simulink library "generallib"  (R2024b)
settings: Solver=VariableStepAuto  StartTime=0.0  StopTime=10.0  RelTol=1e-3
Description:
  | Simulink library with commonly used blocks for
  | Robotics, Vision and Control - 3rd Edition
settings Model: Creator=rpill  LastModifiedBy=pic
settings SolverCC: MaxZcPerStep=1
settings DebuggingCC: UnconnectedInputMsg=warning  UnconnectedOutputMsg=warning  UnconnectedLineMsg=warning
settings ModelReferenceCC: EnableRefExpFcnMdlSchedulingChecks=on
settings RTWCC: GPUComputeCapability=3.5  DLArmComputeVersion=19.05

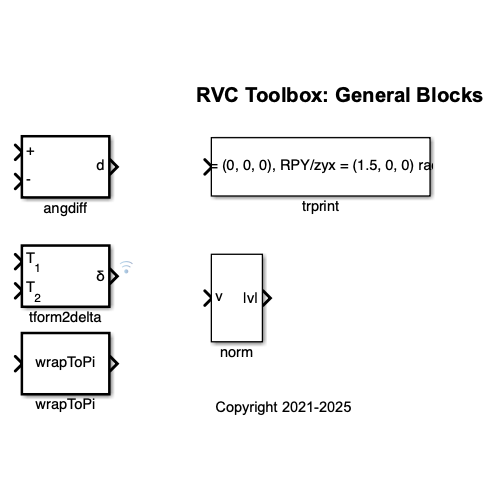
[thumbnail: Simulink's stored preview of the top-level diagram]
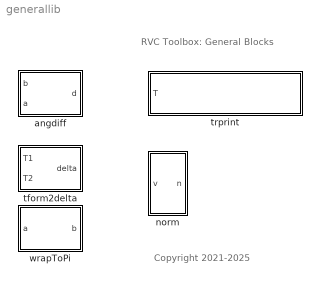
== system generallib ==
  note: Copyright 2021-2025
  note: RVC Toolbox: General Blocks
  angdiff : MATLAB Function  TreatAsAtomicUnit=on
  norm : Subsystem
      mask Display:
      | port_label('output', 1, '|v|', 'texmode', 'on')
      | port_label('input', 1, 'v')
  tform2delta : MATLAB Function  TreatAsAtomicUnit=on
  trprint : Subsystem  mask{options={}}
      mask prompts: options "Options (cell array)"
      mask Display: disp('t = (0, 0, 0), RPY/zyx = (1.5, 0, 0) rad');
  wrapToPi : MATLAB Function  TreatAsAtomicUnit=on

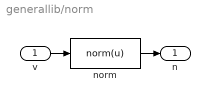
== system generallib/norm ==
  v : Inport
  norm : MATLABFcn  MATLABFcn=norm(u)
  n : Outport  VectorParamsAs1DForOutWhenUnconnected=off
  wires:
  v/1 -> norm/1
  norm/1 -> n/1

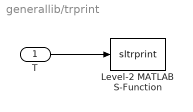
== system generallib/trprint ==
  T : Inport
  Level-2 MATLAB S-Function : M-S-Function  FunctionName=sltrprint  Parameters=options
      mask Display: disp('t = (1.6, -1.3, -1.44), RPY/zyx = (-0.361, -0.181, -0.619) rad');
  wires:
  T/1 -> Level-2 MATLAB S-Function/1

== matlab function generallib/angdiff ==
  data: b input; d output; a input
function d = angdiff(b,a)

d = angdiff(a,b);

end

== matlab function generallib/wrapToPi ==
  data: b output; a input
function b = wrapToPi(a)

b = wrapToPi(a);

end

== matlab function generallib/tform2delta ==
  data: T1 input; delta output; T2 input
function delta = tr2delta(T1,T2)

delta = tform2delta(T1,T2,fliptr=true)';

end
